simulink model "model1"  (R2024b)
settings: Solver=VariableStepAuto  StartTime=0.0  StopTime=10.0  RelTol=1e-3
settings Model: Creator=mehmetcanevi  LastModifiedBy=mehmetcanevi

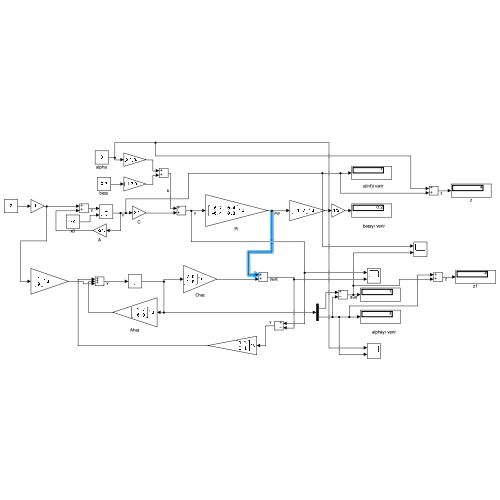
[thumbnail: Simulink's stored preview of the top-level diagram]
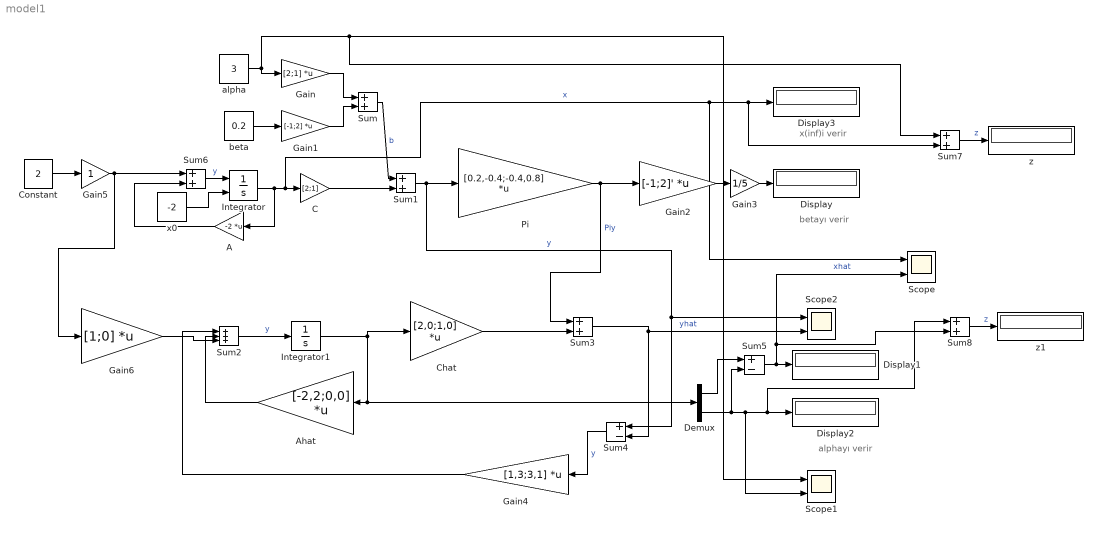
== system model1 ==
  note: betayı verir
  note: x(inf)i verir
  note: alphayı verir
  A : Gain  Gain=-2  Multiplication=Matrix(K*u)
  Ahat : Gain  Gain=[-2,2;0,0]  Multiplication=Matrix(K*u)
  C : Gain  Gain=[2;1]
  Chat : Gain  Gain=[2,0;1,0]  Multiplication=Matrix(K*u)
  Constant : Constant  Value=2
  Demux : Demux  Outputs=2
  Display{,1..3} (4 alike) : Display
  Gain : Gain  Gain=[2;1]  Multiplication=Matrix(K*u)
  Gain1 : Gain  Gain=[-1;2]  Multiplication=Matrix(K*u)
  Gain2 : Gain  Gain=[-1;2]'  Multiplication=Matrix(K*u)
  Gain3 : Gain  Gain=1/5
  Gain4 : Gain  Gain=[1,3;3,1]  Multiplication=Matrix(K*u)
  Gain5 : Gain
  Gain6 : Gain  Gain=[1;0]  Multiplication=Matrix(K*u)
  Integrator : Integrator  InitialConditionSource=external
  Integrator1 : Integrator
  Pi : Gain  Gain=[0.2,-0.4;-0.4,0.8]  Multiplication=Matrix(K*u)
  Scope : Scope  NumInputPorts=2
  Scope1 : Scope  NumInputPorts=2
  Scope2 : Scope  NumInputPorts=2
  Sum{,1,3,6..8} (6 alike) : Sum
  Sum2 : Sum  Inputs=+++
  Sum4 : Sum  Inputs=+-
  Sum5 : Sum  Inputs=+-
  alpha : Constant  Value=3
  beta : Constant  Value=0.2
  x0 : Constant  Value=-2
  z : Display
  z1 : Display
  wires:
  A/1 -> Sum6/2
  x0/1 -> Integrator/2
  Integrator/1 -> Sum7/2, Display3/1, Scope/1, C/1, A/1  "x"
  beta/1 -> Gain1/1
  Gain/1 -> Sum/1
  Gain1/1 -> Sum/2
  C/1 -> Sum1/2
  Sum/1 -> Sum1/1  "b"
  Sum1/1 -> Scope2/1, Sum4/1, Pi/1  "y"
  Pi/1 -> Sum3/1, Gain2/1  "Piy"
  Gain2/1 -> Gain3/1
  Gain3/1 -> Display/1
  Integrator1/1 -> Chat/1, Demux/1, Ahat/1
  Sum2/1 -> Integrator1/1  "y"
  Ahat/1 -> Sum2/2
  Chat/1 -> Sum3/2
  Sum4/1 -> Gain4/1  "y"
  Gain4/1 -> Sum2/1
  Sum3/1 -> Scope2/2, Sum4/2  "yhat"
  Demux/2 -> Scope1/2, Sum8/1, Display2/1, Sum5/2
  Sum5/1 -> Sum8/2, Scope/2, Display1/1  "xhat"
  Demux/1 -> Sum5/1
  Sum6/1 -> Integrator/1  "y"
  Gain5/1 -> Gain6/1, Sum6/1
  Constant/1 -> Gain5/1
  alpha/1 -> Gain/1, Sum7/1, Scope1/1
  Gain6/1 -> Sum2/3
  Sum7/1 -> z/1  "z"
  Sum8/1 -> z1/1  "z"
